simulink model "winda5"  (R2015b)
settings: Solver=FixedStepAuto  StartTime=0.0  StopTime=150  FixedStep=1e-3  RelTol=1e-3
undefined symbols (not defined in the file): sigbuilder_block
libraries: simulink x12
settings Model: Creator=lukinowy  LastModifiedBy=lukinowy

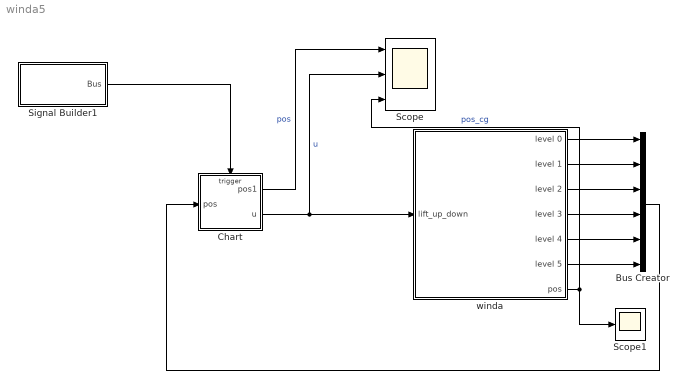
== system winda5 ==
  Bus Creator : BusCreator  Inputs=6
  Chart : Stateflow chart  TreatAsAtomicUnit=on
  Scope : Scope  NumInputPorts=3
  Scope1 : Scope
  Signal Builder1 : Subsystem  Tag=STV Subsys  LoadFcn=sigbuilder_block('load',[56.25 144 498 368.25 ]);  StartFcn=sigbuilder_block('start');  StopFcn=sigbuilder_block('stop');  ClipboardFcn=sigbuilder_block('clipboard');  mask(Sigbuilder block){}
      mask help: Simulink:masks:SigbuilderBlock_MD
      mask init:
      | if ~strcmp(get_param(bdroot(gcbh),'SimulationStatus'),'stopped') tuvar = sigbuilder_block('maskInit'); end
      settings: CopyFcn=sigbuilder_block('copy');  DeleteFcn=sigbuilder_block('delete');  ModelCloseFcn=sigbuilder_block('modelClose');  PreSaveFcn=sigbuilder_block('preSave');  PauseFcn=sigbuilder_block('pause');  ContinueFcn=sigbuilder_block('continue');  NameChangeFcn=sigbuilder_block('namechange');  OpenFcn=sigbuilder_block('open',[56.25 121.5 505.5 369.75 ]);  CloseFcn=sigbuilder_block('close');
      mask Display: plot(0, 0, 100, 100,[2, 2, 32, 32, 2], [68, 8, 8, 68, 68],[32, 2], [38, 38], [32, 19, 2],[53, 60, 44], [32, 17, 17, 2],[16, 16, 31, 31]);txt = getActiveGroup(gcbh);text(2, 100, txt,'verticalAlignment', 'top');
  winda : Subsystem
  wires:
  winda/1(level 0) -> Bus Creator/1
  winda/2(level 1) -> Bus Creator/2
  winda/3(level 2) -> Bus Creator/3
  winda/4(level 3) -> Bus Creator/4
  winda/5(level 4) -> Bus Creator/5
  winda/6(level 5) -> Bus Creator/6
  Bus Creator/1 -> Chart/1(pos)
  Signal Builder1/1(Bus) -> Chart/Trigger
  Chart/2(u) -> Scope/2, winda/1(lift_up_down)  "u"
  Chart/1(pos1) -> Scope/1  "pos"
  winda/7(pos) -> Scope/3, Scope1/1  "pos_cg"

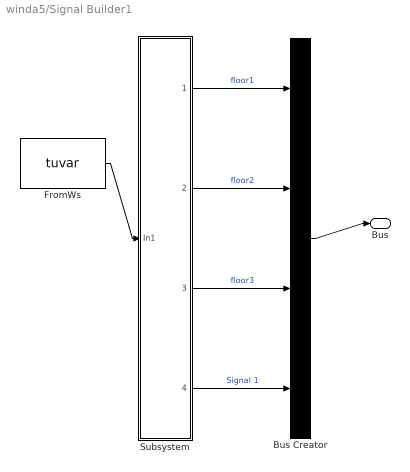
== system winda5/Signal Builder1 ==
  Bus Creator : BusCreator  Tag=Bus Creator  Inputs=4
  FromWs : FromWorkspace  Tag=STV FromWs  VariableName=tuvar  SampleTime=0
      SigBuilderData=|
      | common.afterFinalStr = 'Extrapolate'
      | common.sampleTime = 0
      | dataSet.timeRange = [0 150]
      | dataSet.name = 'Group 1'
      | sbobj.Groups.Name = 'Group 1'
      | sbobj.Groups.Signals(1).Name = 'floor1'
      | sbobj.Groups.Signals(1).XData = [0 61.5 61.5 72.5 72.5 150]
      | sbobj.Groups.Signals(1).YData = [0 0 1.1 1.1 0 0]
      | sbobj.Groups.Signals(2).Name = 'floor2'
      | sbobj.Groups.Signals(2).XData = [0 18 18 22.4 22.4 78.5 78.5 84 84 150]
      | sbobj.Groups.Signals(2).YData = [-1.1 -1.1 1.7 1.7 -1.1 -1.1 1.7 1.7 -1.1 -1.1]
      | sbobj.Groups.Signals(3).Name = 'floor3'
      | sbobj.Groups.Signals(3).XData = [0 1.66666666667 42.5 42.5 52.4 52.4 64.2 64.2 70.8 70.8 150]
      | sbobj.Groups.Signals(3).YData = [0 0 0 2.9 2.9 0 0 2.9 2.9 0 0]
      | sbobj.Groups.Signals(4).Name = 'Signal 1'
      | sbobj.Groups.Signals(4).XData = [0 0.05 0.05 0.1 0.1 0.15 0.15 0.2 0.2 0.25 0.25 0.3 ... (6000 elements, 1x6000)]
      | sbobj.Groups.Signals(4).YData = [2 2 0 0 2 2 0 0 2 2 0 0 ... (6000 elements, 1x6000)]
      | sbobj.Groups.TimeRange = [0 150]
  Subsystem : Subsystem
  Bus : Outport
  wires:
  FromWs/1 -> Subsystem/1(In1)
  Subsystem/1(floor1) -> Bus Creator/1  "floor1"
  Subsystem/2(floor2) -> Bus Creator/2  "floor2"
  Subsystem/3(floor3) -> Bus Creator/3  "floor3"
  Subsystem/4(Signal 1) -> Bus Creator/4  "Signal 1"
  Bus Creator/1 -> Bus/1

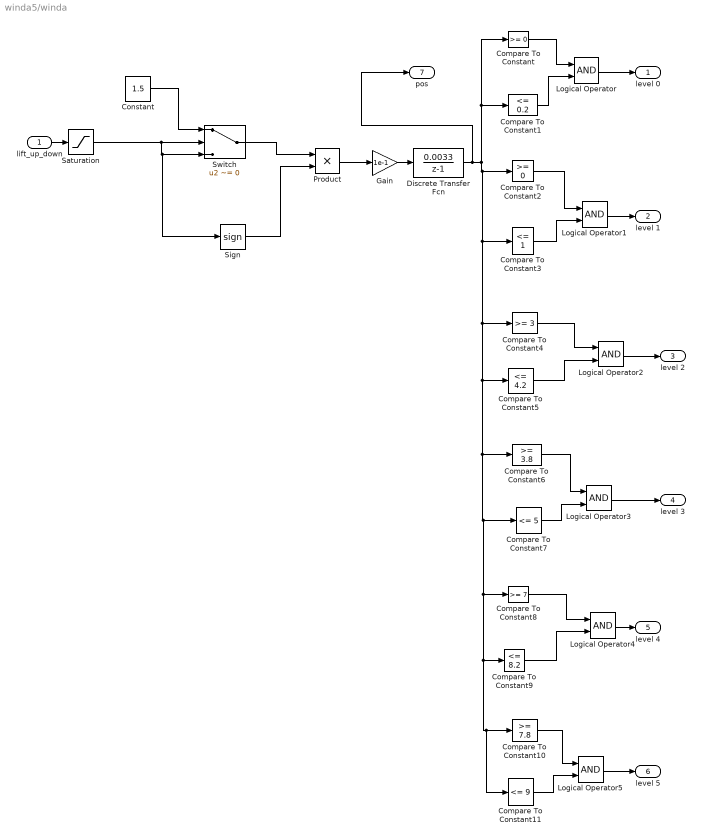
== system winda5/winda ==
  lift_up_down : Inport
  Compare To Constant : simulink/Logic and Bit Operations/Compare To Constant  relop=>=  const=0  OutDataTypeStr=boolean
  Compare To Constant1 : simulink/Logic and Bit Operations/Compare To Constant  relop=<=  const=0.2  OutDataTypeStr=boolean
  Compare To Constant10 : simulink/Logic and Bit Operations/Compare To Constant  relop=>=  const=7.8  OutDataTypeStr=boolean
  Compare To Constant11 : simulink/Logic and Bit Operations/Compare To Constant  relop=<=  const=9  OutDataTypeStr=boolean
  Compare To Constant2 : simulink/Logic and Bit Operations/Compare To Constant  relop=>=  const=0  OutDataTypeStr=boolean
  Compare To Constant3 : simulink/Logic and Bit Operations/Compare To Constant  relop=<=  const=1  OutDataTypeStr=boolean
  Compare To Constant4 : simulink/Logic and Bit Operations/Compare To Constant  relop=>=  const=3  OutDataTypeStr=boolean
  Compare To Constant5 : simulink/Logic and Bit Operations/Compare To Constant  relop=<=  const=4.2  OutDataTypeStr=boolean
  Compare To Constant6 : simulink/Logic and Bit Operations/Compare To Constant  relop=>=  const=3.8  OutDataTypeStr=boolean
  Compare To Constant7 : simulink/Logic and Bit Operations/Compare To Constant  relop=<=  const=5  OutDataTypeStr=boolean
  Compare To Constant8 : simulink/Logic and Bit Operations/Compare To Constant  relop=>=  const=7  OutDataTypeStr=boolean
  Compare To Constant9 : simulink/Logic and Bit Operations/Compare To Constant  relop=<=  const=8.2  OutDataTypeStr=boolean
  Constant : Constant  Value=1.5
  Discrete Transfer Fcn : DiscreteTransferFcn  Numerator=[0.0033]  Denominator=[1 -1]
  Gain : Gain  Gain=1e-1
  Logical Operator{,1..5} (6 alike) : Logic  AllPortsSameDT=off  OutDataTypeStr=boolean
  Product : Product
  Saturation : Saturate  UpperLimit=1  LowerLimit=-1
  Sign : Signum
  Switch : Switch  Criteria=u2 ~= 0
  level 0 : Outport
  level 1 : Outport  Port=2
  level 2 : Outport  Port=3
  level 3 : Outport  Port=4
  level 4 : Outport  Port=5
  level 5 : Outport  Port=6
  pos : Outport  Port=7
  wires:
  Saturation/1 -> Sign/1, Switch/3, Switch/2
  Gain/1 -> Discrete Transfer Fcn/1
  lift_up_down/1 -> Saturation/1
  Discrete Transfer Fcn/1 -> pos/1, Compare To Constant11/1, Compare To Constant10/1, Compare To Constant9/1, Compare To Constant8/1, Compare To Constant7/1, Compare To Constant6/1, Compare To Constant5/1, Compare To Constant4/1, Compare To Constant3/1, Compare To Constant2/1, Compare To Constant1/1, Compare To Constant/1
  Constant/1 -> Switch/1
  Sign/1 -> Product/2
  Switch/1 -> Product/1
  Product/1 -> Gain/1
  Compare To Constant/1 -> Logical Operator/1
  Compare To Constant1/1 -> Logical Operator/2
  Compare To Constant2/1 -> Logical Operator1/1
  Compare To Constant3/1 -> Logical Operator1/2
  Compare To Constant4/1 -> Logical Operator2/1
  Compare To Constant5/1 -> Logical Operator2/2
  Compare To Constant6/1 -> Logical Operator3/1
  Compare To Constant7/1 -> Logical Operator3/2
  Compare To Constant8/1 -> Logical Operator4/1
  Compare To Constant9/1 -> Logical Operator4/2
  Compare To Constant10/1 -> Logical Operator5/1
  Compare To Constant11/1 -> Logical Operator5/2
  Logical Operator/1 -> level 0/1
  Logical Operator1/1 -> level 1/1
  Logical Operator2/1 -> level 2/1
  Logical Operator3/1 -> level 3/1
  Logical Operator4/1 -> level 4/1
  Logical Operator5/1 -> level 5/1

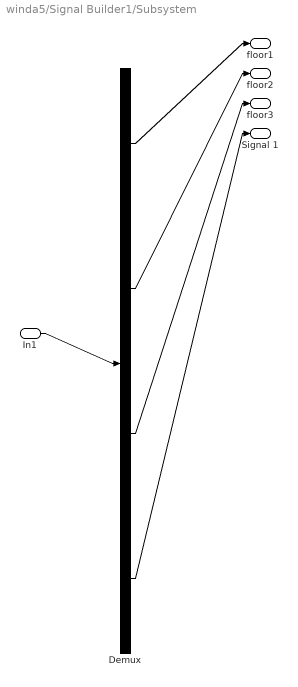
== system winda5/Signal Builder1/Subsystem ==
  In1 : Inport
  Demux : Demux  Tag=STV Demux
  floor1 : Outport  Tag=STV Outport
  floor2 : Outport  Tag=STV Outport  Port=2
  floor3 : Outport  Tag=STV Outport  Port=3
  Signal 1 : Outport  Tag=STV Outport  Port=4
  wires:
  Demux/1 -> floor1/1
  Demux/2 -> floor2/1
  Demux/3 -> floor3/1
  Demux/4 -> Signal 1/1
  In1/1 -> Demux/1

== stateflow chart winda5/Chart ==
  state LICZNIK [parallel]
    on clk:
    i = i+1;
    if (i==10)
    i=uint32(0);
    sek=sek+1;
    end
    on rst:
    i=uint32(0);
    sek=uint16(0);
    settings: executionOrder=1
  state POZYCJA [parallel]
    en: pos1=uint8(1);
    on clk:
    if  all(pos(1:2)==[1 1])
    pos1 = uint8(1);
    dwa = logical(1);
    elseif all(pos(3:4) == [1 1])
    pos1 = uint8(2);
    dwa = logical(1);
    elseif all(pos(5:6) == [1 1])
    pos1 = uint8(3);
    dwa = logical(1);
    else dwa=logical(0);
    end
    settings: executionOrder=2
  state STEROWANIE [parallel]
    settings: executionOrder=3
    state PAUSE
      en:
      rst;
      u=int8(0);
      on clk:
      if sek>5
      wznow;
      end
    state UP
      en:
      u=int8(1);
    state WAIT
      en:
      rst;
      u=int8(0);
      if k~=pos1 || ~dwa
      start;
      end
      on clk:
      if k==int8(3)
      dk=int8(-1);
      elseif k==int8(1)
      dk=int8(1);
      end
      k=k+dk;
      if kolejka(k)==int8(1)
      start;
      end
    state DOWN
      en:
      u=int8(-1);
    state TIMEOUT
      en:
      u=int8(-1);
      kolejka(1)=1;
    DOWN -> PAUSE : zatrzymaj
    UP -> PAUSE : zatrzymaj
    PAUSE -> WAIT : wznow
    WAIT -> UP [order 1] : start [k>=pos1]
    WAIT -> DOWN [order 2] : start [k<pos1]
    TIMEOUT -> WAIT [order 2] : zatrzymaj {u=int8(0); k=int8(pos1);}
    WAIT -> TIMEOUT [order 3] : [sek>5 && pos1~=1]
    (default) -> WAIT
    TIMEOUT -> WAIT [order 1] : floor1 {k= int8(1)}
    TIMEOUT -> WAIT [order 4] : floor3 {k= int8(3)}
    TIMEOUT -> WAIT [order 3] : floor2 {k= int8(2)}
  state ZATRZYMAC [parallel]
    on clk:
    if kolejka(pos1)==1 && dwa
    kolejka(pos1)=0;
    zatrzymaj;
    end
    settings: executionOrder=5
  state ZGLOSZENIA [parallel]
    on floor1: kolejka(1)=1;
    on floor2: kolejka(2)=1;
    on floor3: kolejka(3)=1;
    settings: executionOrder=4
  data: i local uint32 =uint32(0); sek local uint16 =uint16(0); pos input boolean size=[1 6]; pos1 output uint8 =uint8(1); kolejka local uint8 size=[1 3] =uint8([1 0 0]); u output int8 =int8(0); dwa local boolean =logical(0); k local int8 =int8(1); dk local int8 =int8(1)
  events: rst local FUNCTION_CALL_EVENT; zatrzymaj local FUNCTION_CALL_EVENT; wznow local FUNCTION_CALL_EVENT; floor1 input RISING_EDGE_EVENT; floor2 input RISING_EDGE_EVENT; floor3 input RISING_EDGE_EVENT; clk input RISING_EDGE_EVENT; start local FUNCTION_CALL_EVENT
